simulink model "Hoisting"  (R2021a)
settings: Solver=VariableStepAuto  StartTime=0.0  StopTime=10.0  RelTol=1e-3
values from neighbouring files (symbols this model uses):
  Fhb_max = Thb_max/rhd    (= 66666.6666667)    [Data.m]
  g = 9.80665    [Data.m]
undefined symbols (not defined in the file or in its folder): gear, Mh, ml, rd, theta0, w0
settings Model: Creator=jpss8  LastModifiedBy=jpss8

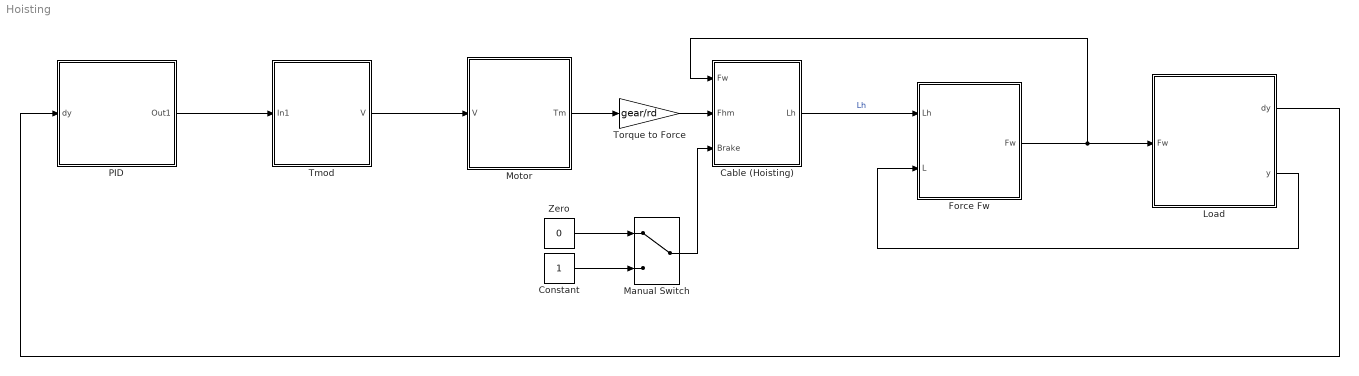
== system Hoisting ==
  Cable (Hoisting) : Subsystem
  Constant : Constant
  Force Fw : Subsystem
  Load : Subsystem
  Manual Switch : ManualSwitch
  Motor : Subsystem
  PID : Subsystem
  Tmod : Subsystem
  Torque to Force : Gain  Gain=gear/rd
  Zero : Constant  Value=0  OutDataTypeStr=Inherit: Inherit via back propagation
  wires:
  Force Fw/1(Fw) -> Cable (Hoisting)/1(Fw), Load/1(Fw)
  Cable (Hoisting)/1(Lh) -> Force Fw/1(Lh)  "Lh"
  Torque to Force/1 -> Cable (Hoisting)/2(Fhm)
  Manual Switch/1 -> Cable (Hoisting)/3(Brake)
  Zero/1 -> Manual Switch/1
  Constant/1 -> Manual Switch/2
  PID/1(Out1) -> Tmod/1(In1)
  Load/1(dy) -> PID/1(dy)
  Motor/1(Tm) -> Torque to Force/1
  Load/2(y) -> Force Fw/2(L)
  Tmod/1(V) -> Motor/1(V)

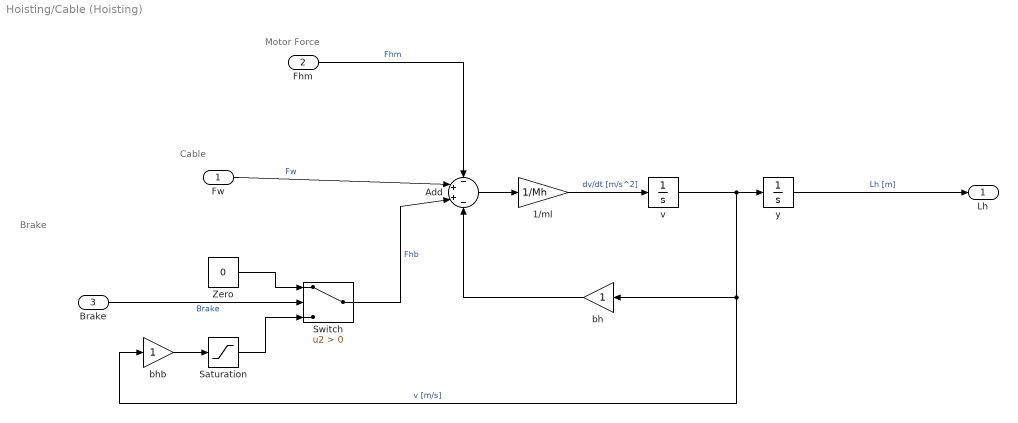
== system Hoisting/Cable (Hoisting) ==
  note: Motor Force
  note: Cable
  note: Brake
  Fw : Inport
  Fhm : Inport  Port=2
  Brake : Inport  Port=3
  1/ml : Gain  Gain=1/Mh
  Add : Sum  Inputs=-++-
  Saturation : Saturate  UpperLimit=Fhb_max  LowerLimit=-Fhb_max
  Switch : Switch  Criteria=u2 > Threshold
  Zero : Constant  Value=0  OutDataTypeStr=Inherit: Inherit via back propagation
  bh : Gain
  bhb : Gain
  v : Integrator  InitialCondition=w0
  y : Integrator  InitialCondition=theta0
  Lh : Outport
  wires:
  Fw/1 -> Add/2  "Fw"
  v/1 -> bhb/1, bh/1, y/1  "v [m/s]"
  y/1 -> Lh/1  "Lh [m]"
  Fhm/1 -> Add/1  "Fhm"
  1/ml/1 -> v/1  "dv/dt [m/s^2]"
  Add/1 -> 1/ml/1
  bh/1 -> Add/4
  Switch/1 -> Add/3  "Fhb"
  Brake/1 -> Switch/2  "Brake"
  Zero/1 -> Switch/1
  bhb/1 -> Saturation/1
  Saturation/1 -> Switch/3

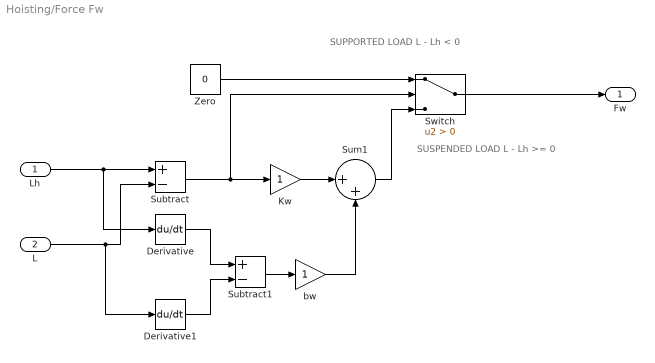
== system Hoisting/Force Fw ==
  note: SUPPORTED LOAD L - Lh < 0
  note: SUSPENDED LOAD L - Lh >= 0
  Lh : Inport
  L : Inport  Port=2
  Derivative : Derivative
  Derivative1 : Derivative
  Kw : Gain
  Subtract : Sum  Inputs=+-
  Subtract1 : Sum  Inputs=+-
  Sum1 : Sum  Inputs=|++
  Switch : Switch  Criteria=u2 > Threshold
  Zero : Constant  Value=0  OutDataTypeStr=Inherit: Inherit via back propagation
  bw : Gain
  Fw : Outport
  wires:
  Lh/1 -> Subtract/1, Derivative/1
  L/1 -> Derivative1/1, Subtract/2
  Derivative/1 -> Subtract1/1
  Derivative1/1 -> Subtract1/2
  Subtract/1 -> Kw/1, Switch/2
  Zero/1 -> Switch/1
  Sum1/1 -> Switch/3
  Kw/1 -> Sum1/1
  Subtract1/1 -> bw/1
  Switch/1 -> Fw/1
  bw/1 -> Sum1/2

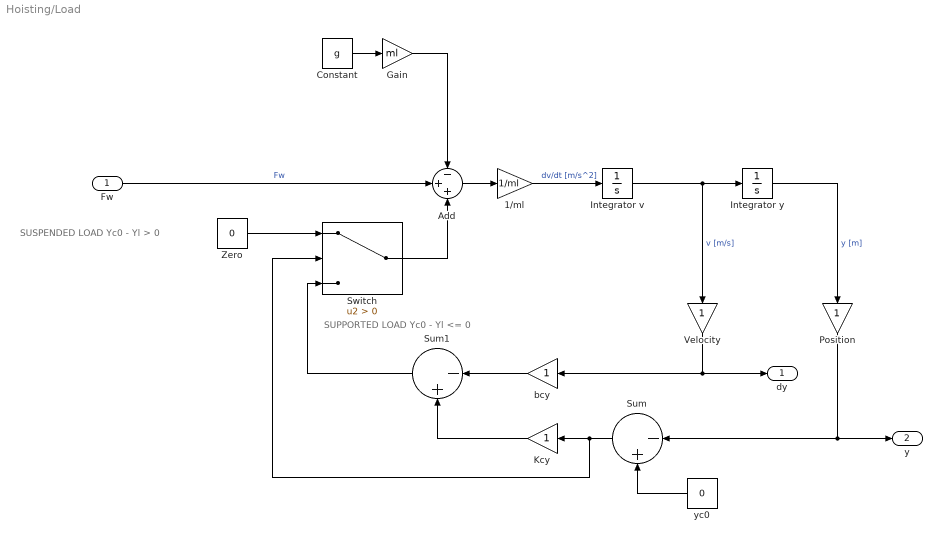
== system Hoisting/Load ==
  note: SUPPORTED LOAD Yc0 - Yl <= 0
  note: SUSPENDED LOAD Yc0 - Yl > 0
  Fw : Inport
  1/ml : Gain  Gain=1/ml
  Add : Sum  Inputs=-++
  Constant : Constant  Value=g
  Gain : Gain  Gain=ml
  Integrator v : Integrator  InitialCondition=w0
  Integrator y : Integrator  InitialCondition=theta0
  Kcy : Gain
  Position : Gain
  Sum : Sum  Inputs=|-+
  Sum1 : Sum  Inputs=|-+
  Switch : Switch  Criteria=u2 > Threshold
  Velocity : Gain
  Zero : Constant  Value=0  OutDataTypeStr=Inherit: Inherit via back propagation
  bcy : Gain
  yc0 : Constant  Value=0  OutDataTypeStr=Inherit: Inherit via back propagation
  dy : Outport
  y : Outport  Port=2
  wires:
  Constant/1 -> Gain/1
  Integrator y/1 -> Position/1  "y [m]"
  Add/1 -> 1/ml/1
  1/ml/1 -> Integrator v/1  "dv/dt [m/s^2]"
  Integrator v/1 -> Velocity/1, Integrator y/1  "v [m/s]"
  Fw/1 -> Add/2  "Fw"
  Position/1 -> Sum/1, y/1
  yc0/1 -> Sum/2
  Sum/1 -> Switch/2, Kcy/1
  Velocity/1 -> dy/1, bcy/1
  Kcy/1 -> Sum1/2
  bcy/1 -> Sum1/1
  Switch/1 -> Add/3
  Gain/1 -> Add/1
  Zero/1 -> Switch/1
  Sum1/1 -> Switch/3

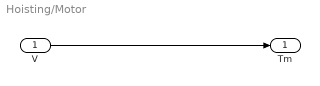
== system Hoisting/Motor ==
  V : Inport
  Tm : Outport
  wires:
  V/1 -> Tm/1

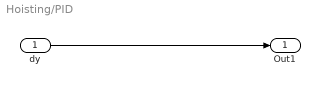
== system Hoisting/PID ==
  dy : Inport
  Out1 : Outport
  wires:
  dy/1 -> Out1/1

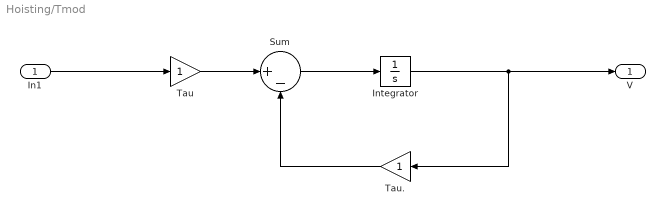
== system Hoisting/Tmod ==
  In1 : Inport
  Integrator : Integrator
  Sum : Sum  Inputs=|+-
  Tau : Gain
  Tau. : Gain
  V : Outport
  wires:
  In1/1 -> Tau/1
  Tau/1 -> Sum/1
  Sum/1 -> Integrator/1
  Tau./1 -> Sum/2
  Integrator/1 -> Tau./1, V/1
